simulink model "AWGN_detect_ID"  (Simulink 7.5)
settings: Solver=FixedStepDiscrete  SolverMode=SingleTasking  StartTime=0.0  StopTime=1  FixedStep=1/100000  RelTol=1e-3
libraries: commchan3 x1, commsink2 x1, commfilt2 x1, commrandsrc2 x1
settings Model: Creator=amoura  LastModifiedBy=hsalgado
settings DataIOCC: LimitDataPoints=off  SignalLoggingName=sigsOut
settings OptimizationCC: BooleanDataType=off  InitFltsAndDblsToZero=on
settings DebuggingCC: SaveWithParameterizedLinksMsg=none  SignalResolutionControl=TryResolveAllWithWarning  SolverPrmCheckMsg=none  MultiTaskDSMMsg=warning  MultiTaskCondExecSysMsg=none  StrictBusMsg=None
settings HardwareCC: TargetUnknown=on
settings RTWCC: TemplateMakefile=grt_unix.tmf  IncludeERTFirstTime=on
settings GRTTargetCC: TargetFcnLib=ansi_tfl_tmw.mat  ModelReferenceCompliant=off  MatFileLogging=off

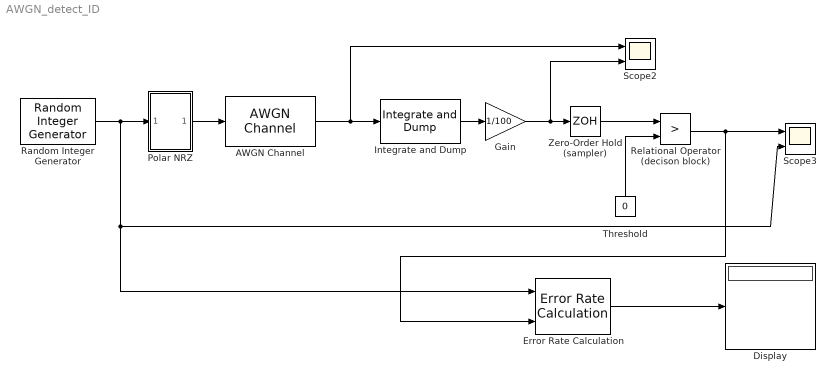
== system AWGN_detect_ID ==
  AWGN Channel : commchan3/AWGN Channel  SystemSampleTime=-1  seed=67  noiseMode=Variance from mask  EbNodB=10  EsNodB=10  SNRdB=10  bitsPerSym=1  Ps=1  Tsym=1  variance=160
  Display : Display
  Error Rate Calculation : commsink2/Error Rate Calculation  N=1  st_delay=0  cp_mode=Entire frame  subframe=[]  PMode=Port  WsName=ErrorVec  RsMode2=off  stop=off  numErr=100  maxBits=1e6
  Gain : Gain  Gain=1/100  RndMeth=Nearest  SampleTime=1/100000  SaturateOnIntegerOverflow=on  OutDataTypeStr=Inherit: Same as input  ParamDataTypeStr=Inherit: Same as input
  Integrate and Dump : commfilt2/Integrate and Dump  DialogController=commDDGCreate  DialogControllerArgs=DataTag1  obssamples=100  offsetsamples=1  nodump=on  roundingMode=Floor  overflowMode=off
  Polar NRZ : Subsystem
      mask Type: Polar NRZ
      mask Description:
      | This block encodes a unipolar NRZ signal into the polar NRZ line code
      | 
      | The output values are +1 for a nonzero input and -1 for a zero one.
      mask Display: disp('Polar\nNRZ')
  Random Integer Generator : commrandsrc2/Random Integer Generator  SystemSampleTime=-1  mul=2  seed=37  Ts=1/1000  frameBased=off  sampPerFrame=1  orient=off  outDataType=double
  Relational Operator (decison block) : RelationalOperator  Operator=>  InputSameDT=on
  Scope2 : Scope  NumInputPorts=2
      settings: TickLabels=on  YMin=-5~-5  YMax=5~5  DataFormat=Array
  Scope3 : Scope  NumInputPorts=2
      settings: TickLabels=on  YMin=-5~-5  YMax=5~5  DataFormat=Array  SampleInput=on  SampleTime=1/1000
  Threshold : Constant  Value=0
  Zero-Order Hold (sampler) : ZeroOrderHold  SampleTime=1/1000
  wires:
  Integrate and Dump/1 -> Gain/1
  Random Integer Generator/1 -> Error Rate Calculation/1, Scope3/2, Polar NRZ/1(In1)
  Polar NRZ/1(Out1) -> AWGN Channel/1
  AWGN Channel/1 -> Scope2/1, Integrate and Dump/1
  Error Rate Calculation/1 -> Display/1
  Relational Operator (decison block)/1 -> Error Rate Calculation/2, Scope3/1
  Zero-Order Hold (sampler)/1 -> Relational Operator (decison block)/1
  Threshold/1 -> Relational Operator (decison block)/2
  Gain/1 -> Zero-Order Hold (sampler)/1, Scope2/2

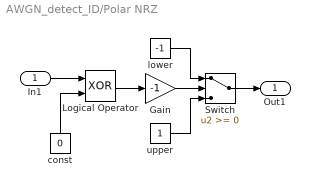
== system AWGN_detect_ID/Polar NRZ ==
  In1 : Inport
  Gain : Gain  Gain=-1  SaturateOnIntegerOverflow=on  OutDataTypeStr=Inherit: Same as input  ParamDataTypeStr=Inherit: Same as input
  Logical Operator : Logic  Operator=XOR
  Switch : Switch  SaturateOnIntegerOverflow=on  InputSameDT=on
  const : Constant  Value=0
  lower : Constant  Value=-1
  upper : Constant
  Out1 : Outport
  wires:
  const/1 -> Logical Operator/2
  Logical Operator/1 -> Gain/1
  Switch/1 -> Out1/1
  Gain/1 -> Switch/2
  upper/1 -> Switch/3
  lower/1 -> Switch/1
  In1/1 -> Logical Operator/1
